simulink model "momentumBasedFlying"  (Simulink 10.2)
settings: Solver=FixedStepAuto  StartTime=0.0  StopTime=Config.simulationTime  FixedStep=Config.tStep  RelTol=1e-3
InitFcn:
  | cd(fileparts(which(bdroot)));
  | initMomentumBasedFlying;
StopFcn:
  | cd(fileparts(which(bdroot)));
  | stopMomentumBasedFlying;
undefined symbols (not defined in the file or in its folder): aerodynamics_config, biasVectorConstraint_feet, Config, confVisualizer, ConstraintMatrix_feet, DiscIntNeverNeededParam, jets_config
libraries: WBToolboxLibrary x85
(part 3 of 4)

== system momentumBasedFlying/iRonCub/Forward Dynamics/old_simulator_subsystem/Compute generalized external wrench and jet thrust/Compute generalized jet wrench ==
  <J_jets> : Inport
  <matrixOfJetAxes> : Inport  Port=2
  jets_input : Inport  Port=3
  Discrete-Time Integrator : DiscreteIntegrator  InitialCondition=Config.initialConditions.jets_thrust  SampleTime=-1  ICPrevOutput=DiscIntNeverNeededParam  ICPrevScaledInput=DiscIntNeverNeededParam
  Discrete-Time Integrator1 : DiscreteIntegrator  SampleTime=-1  ICPrevOutput=DiscIntNeverNeededParam  ICPrevScaledInput=DiscIntNeverNeededParam
  J^T*f : Product  Multiplication=Matrix(*)
  Jet Dynamics : MATLAB Function  TreatAsAtomicUnit=on
  Transpose : Math  Operator=transpose  SignedPower=on  SaturateOnIntegerOverflow=on
  "compute_jet_wrenches " : MATLAB Function  TreatAsAtomicUnit=on
  generalized_jet_wrench : Outport  VectorParamsAs1DForOutWhenUnconnected=off
  jet_intensities : Outport  Port=2  VectorParamsAs1DForOutWhenUnconnected=off
  wires:
  "compute_jet_wrenches "/1(wrenches_vector) -> J^T*f/2  "jet_wrenches_vectors"
  <matrixOfJetAxes>/1 -> "compute_jet_wrenches "/1(matrix_of_jet_axis)
  Transpose/1 -> J^T*f/1  "J_jets_transpose"
  <J_jets>/1 -> Transpose/1
  jets_input/1 -> Jet Dynamics/1(u)
  Discrete-Time Integrator/1 -> jet_intensities/1, "compute_jet_wrenches "/2(jet_intensities), Jet Dynamics/2(jetIntensities)  "jet_intensities"
  J^T*f/1 -> generalized_jet_wrench/1  "generalized_jet_wrench"
  Jet Dynamics/2(jetAccelerationOut) -> Discrete-Time Integrator1/1
  Discrete-Time Integrator1/1 -> Jet Dynamics/3(jetDerivatives)  "jets_velocities"
  Jet Dynamics/1(jetDerivativesOut) -> Discrete-Time Integrator/1

== system momentumBasedFlying/iRonCub/Forward Dynamics/old_simulator_subsystem/Dynamics and Kinematics/Dynamic Quantities ==
  w_H_b : Inport
  w_baseTwist : Inport  Port=2
  jointPos : Inport  Port=3
  jointVel : Inport  Port=4
  GetBiasForces : WBToolboxLibrary/Model/Dynamics/GetBiasForces
      settings: SourceProductName=WholeBodyToolbox
  MassMatrix : WBToolboxLibrary/Model/Dynamics/MassMatrix
      settings: SourceProductName=WholeBodyToolbox
  M : Outport  VectorParamsAs1DForOutWhenUnconnected=off
  "h " : Outport  Port=2  VectorParamsAs1DForOutWhenUnconnected=off
  wires:
  w_H_b/1 -> GetBiasForces/1, MassMatrix/1  "w_H_b"
  w_baseTwist/1 -> GetBiasForces/3
  jointVel/1 -> GetBiasForces/4
  MassMatrix/1 -> M/1
  GetBiasForces/1 -> "h "/1
  jointPos/1 -> GetBiasForces/2, MassMatrix/2

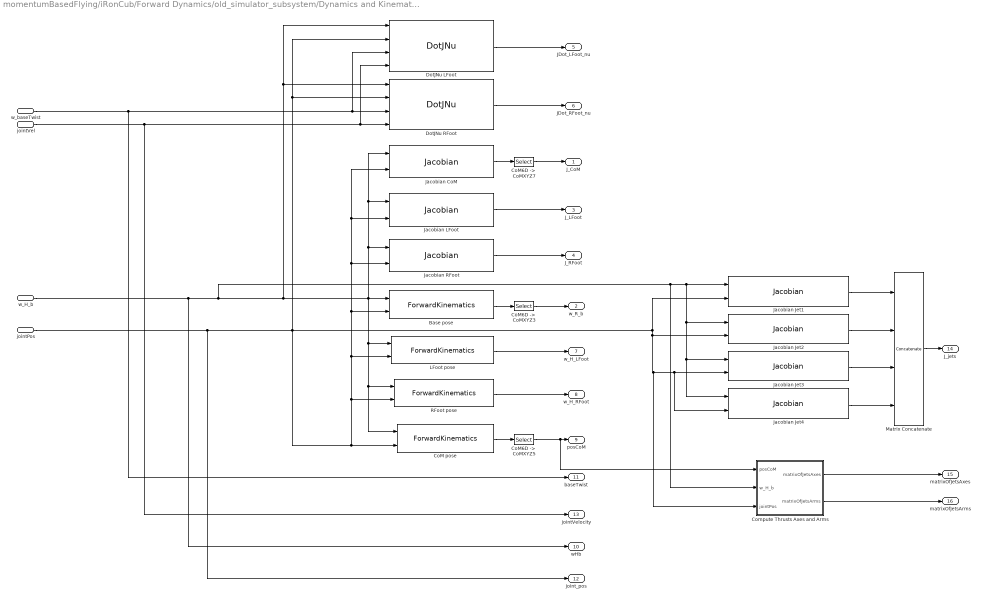
== system momentumBasedFlying/iRonCub/Forward Dynamics/old_simulator_subsystem/Dynamics and Kinematics/Kinematic Quantities ==
  w_H_b : Inport
  w_baseTwist : Inport  Port=2
  jointPos : Inport  Port=3
  jointVel : Inport  Port=4
  Base pose : WBToolboxLibrary/Model/Kinematics/ForwardKinematics  frameName=Frames.BASE_LINK
      settings: SourceProductName=WholeBodyToolbox
  CoM pose : WBToolboxLibrary/Model/Kinematics/ForwardKinematics  frameName=Frames.COM_FRAME
      settings: SourceProductName=WholeBodyToolbox
  "CoM6D ->  CoMXYZ3" : Selector  NumberOfDimensions=2  InputPortWidth=7  IndexOptions=Index vector (dialog),Index vector (dialog)  Indices=[1 2 3],[1 2 3]  OutputSizes=1,1
  "CoM6D ->  CoMXYZ5" : Selector  NumberOfDimensions=2  InputPortWidth=7  IndexOptions=Index vector (dialog),Index vector (dialog)  Indices=[1 2 3],[4]  OutputSizes=1,1
  "CoM6D ->  CoMXYZ7" : Selector  NumberOfDimensions=2  InputPortWidth=7  IndexOptions=Index vector (dialog),Index vector (dialog)  Indices=[1 2 3],[1:6+Config.N_DOF]  OutputSizes=1,1
  Compute Thrusts Axes and Arms : Subsystem
  DotJNu LFoot : WBToolboxLibrary/Model/Jacobians/DotJNu  frameName=Frames.LFOOT_FRAME
      settings: SourceProductName=WholeBodyToolbox
  DotJNu RFoot : WBToolboxLibrary/Model/Jacobians/DotJNu  frameName=Frames.RFOOT_FRAME
      settings: SourceProductName=WholeBodyToolbox
  Jacobian CoM : WBToolboxLibrary/Model/Jacobians/Jacobian  frameName=Frames.COM_FRAME
      settings: SourceProductName=WholeBodyToolbox
  Jacobian Jet1 : WBToolboxLibrary/Model/Jacobians/Jacobian  frameName=Frames.JET1_FRAME
      settings: SourceProductName=WholeBodyToolbox
  Jacobian Jet2 : WBToolboxLibrary/Model/Jacobians/Jacobian  frameName=Frames.JET2_FRAME
      settings: SourceProductName=WholeBodyToolbox
  Jacobian Jet3 : WBToolboxLibrary/Model/Jacobians/Jacobian  frameName=Frames.JET3_FRAME
      settings: SourceProductName=WholeBodyToolbox
  Jacobian Jet4 : WBToolboxLibrary/Model/Jacobians/Jacobian  frameName=Frames.JET4_FRAME
      settings: SourceProductName=WholeBodyToolbox
  Jacobian LFoot : WBToolboxLibrary/Model/Jacobians/Jacobian  frameName=Frames.LFOOT_FRAME
      settings: SourceProductName=WholeBodyToolbox
  Jacobian RFoot : WBToolboxLibrary/Model/Jacobians/Jacobian  frameName=Frames.RFOOT_FRAME
      settings: SourceProductName=WholeBodyToolbox
  LFoot pose : WBToolboxLibrary/Model/Kinematics/ForwardKinematics  frameName=Frames.LFOOT_FRAME
      settings: SourceProductName=WholeBodyToolbox
  Matrix Concatenate : Concatenate  NumInputs=4  Mode=Multidimensional array
  RFoot pose : WBToolboxLibrary/Model/Kinematics/ForwardKinematics  frameName=Frames.RFOOT_FRAME
      settings: SourceProductName=WholeBodyToolbox
  J_CoM : Outport  VectorParamsAs1DForOutWhenUnconnected=off
  w_R_b : Outport  Port=2  VectorParamsAs1DForOutWhenUnconnected=off
  J_LFoot : Outport  Port=3  VectorParamsAs1DForOutWhenUnconnected=off
  J_RFoot : Outport  Port=4  VectorParamsAs1DForOutWhenUnconnected=off
  JDot_LFoot_nu : Outport  Port=5  VectorParamsAs1DForOutWhenUnconnected=off
  JDot_RFoot_nu : Outport  Port=6  VectorParamsAs1DForOutWhenUnconnected=off
  w_H_LFoot : Outport  Port=7  VectorParamsAs1DForOutWhenUnconnected=off
  w_H_RFoot : Outport  Port=8  VectorParamsAs1DForOutWhenUnconnected=off
  posCoM : Outport  Port=9  VectorParamsAs1DForOutWhenUnconnected=off
  wHb : Outport  Port=10
  baseTwist : Outport  Port=11
  joint_pos : Outport  Port=12
  jointVelocity : Outport  Port=13
  J_jets : Outport  Port=14  VectorParamsAs1DForOutWhenUnconnected=off
  matrixOfJetsAxes : Outport  Port=15  VectorParamsAs1DForOutWhenUnconnected=off
  matrixOfJetsArms : Outport  Port=16  VectorParamsAs1DForOutWhenUnconnected=off
  wires:
  CoM pose/1 -> "CoM6D ->  CoMXYZ5"/1
  "CoM6D ->  CoMXYZ3"/1 -> w_R_b/1
  Jacobian CoM/1 -> "CoM6D ->  CoMXYZ7"/1
  Jacobian RFoot/1 -> J_RFoot/1
  Jacobian LFoot/1 -> J_LFoot/1
  DotJNu RFoot/1 -> JDot_RFoot_nu/1
  DotJNu LFoot/1 -> JDot_LFoot_nu/1
  jointVel/1 -> jointVelocity/1, DotJNu RFoot/4, DotJNu LFoot/4
  w_baseTwist/1 -> baseTwist/1, DotJNu LFoot/3, DotJNu RFoot/3
  RFoot pose/1 -> w_H_RFoot/1
  LFoot pose/1 -> w_H_LFoot/1
  Base pose/1 -> "CoM6D ->  CoMXYZ3"/1
  "CoM6D ->  CoMXYZ7"/1 -> J_CoM/1
  Compute Thrusts Axes and Arms/1(matrixOfJetsAxes) -> matrixOfJetsAxes/1
  Compute Thrusts Axes and Arms/2(matrixOfJetsArms) -> matrixOfJetsArms/1
  w_H_b/1 -> Compute Thrusts Axes and Arms/2(w_H_b), Jacobian Jet4/1, Jacobian Jet3/1, Jacobian Jet2/1, Jacobian Jet1/1, DotJNu LFoot/1, DotJNu RFoot/1, Jacobian LFoot/1, Jacobian CoM/1, Jacobian RFoot/1, CoM pose/1, RFoot pose/1, LFoot pose/1, Base pose/1, wHb/1
  Matrix Concatenate/1 -> J_jets/1
  Jacobian Jet3/1 -> Matrix Concatenate/3
  jointPos/1 -> Jacobian Jet4/2, Jacobian Jet3/2, Compute Thrusts Axes and Arms/3(jointPos), Jacobian Jet2/2, Jacobian Jet1/2, LFoot pose/2, Jacobian RFoot/2, Jacobian LFoot/2, Jacobian CoM/2, Base pose/2, RFoot pose/2, CoM pose/2, DotJNu RFoot/2, DotJNu LFoot/2, joint_pos/1
  Jacobian Jet4/1 -> Matrix Concatenate/4
  Jacobian Jet1/1 -> Matrix Concatenate/1
  Jacobian Jet2/1 -> Matrix Concatenate/2
  "CoM6D ->  CoMXYZ5"/1 -> Compute Thrusts Axes and Arms/1(posCoM), posCoM/1

== system momentumBasedFlying/FLYING CONTROLLER (CORE) V2.5/Dynamics and Kinematics/Dynamic Quantities/Momentum and CentroidalMomentum Matrix/CentroidalMomentum Matrix iCub 23/25 DoFs/CMM_base ==
  w_H_b : Inport
  jointPos : Inport  Port=2
  CentroidalMomentum{21..25,31} (6 alike) : WBToolboxLibrary/Model/Dynamics/CentroidalMomentum
      settings: SourceProductName=WholeBodyToolbox
  Constant : Constant  Value=[1,0,0,0,0,0]
  Constant1 : Constant  Value=[0,1,0,0,0,0]
  Constant2 : Constant  Value=zeros(Config.N_DOF,1)
  Constant3 : Constant  Value=[0,0,0,1,0,0]
  Constant37 : Constant  Value=[0,0,1,0,0,0]
  Constant4 : Constant  Value=[0,0,0,0,1,0]
  Constant6 : Constant  Value=[0,0,0,0,0,1]
  Matrix Concatenate : Concatenate  NumInputs=6  Mode=Multidimensional array  ConcatenateDimension=2
  CMM_base : Outport  VectorParamsAs1DForOutWhenUnconnected=off
  wires:
  w_H_b/1 -> CentroidalMomentum31/1, CentroidalMomentum25/1, CentroidalMomentum24/1, CentroidalMomentum23/1, CentroidalMomentum22/1, CentroidalMomentum21/1
  jointPos/1 -> CentroidalMomentum31/2, CentroidalMomentum25/2, CentroidalMomentum24/2, CentroidalMomentum23/2, CentroidalMomentum22/2, CentroidalMomentum21/2
  CentroidalMomentum25/1 -> Matrix Concatenate/5
  Matrix Concatenate/1 -> CMM_base/1
  CentroidalMomentum23/1 -> Matrix Concatenate/3
  CentroidalMomentum24/1 -> Matrix Concatenate/4
  CentroidalMomentum31/1 -> Matrix Concatenate/6
  Constant6/1 -> CentroidalMomentum31/3
  Constant/1 -> CentroidalMomentum21/3
  Constant1/1 -> CentroidalMomentum22/3
  Constant37/1 -> CentroidalMomentum23/3
  Constant2/1 -> CentroidalMomentum21/4, CentroidalMomentum31/4, CentroidalMomentum25/4, CentroidalMomentum24/4, CentroidalMomentum23/4, CentroidalMomentum22/4
  Constant4/1 -> CentroidalMomentum25/3
  Constant3/1 -> CentroidalMomentum24/3
  CentroidalMomentum22/1 -> Matrix Concatenate/2
  CentroidalMomentum21/1 -> Matrix Concatenate/1

== system momentumBasedFlying/FLYING CONTROLLER (CORE) V2.5/Dynamics and Kinematics/Dynamic Quantities/Momentum and CentroidalMomentum Matrix/CentroidalMomentum Matrix iCub 23/25 DoFs/CMM_joints ==
  w_H_b : Inport
  jointPos : Inport  Port=2
  SelMatrix : Inport  Port=3
  CMM Joints Group 1 : Subsystem
  CMM Joints Group 2 : Subsystem
  CMM Joints Group 3 : Subsystem
  CMM Joints Group 4 : Subsystem
  CMM Joints Group 5 : Subsystem
  Matrix Concatenate6 : Concatenate  NumInputs=4  Mode=Multidimensional array  ConcatenateDimension=2
  CMM_joints_from_1_to_20 : Outport  VectorParamsAs1DForOutWhenUnconnected=off
  CMM_group5_25DoFs : Outport  Port=2  VectorParamsAs1DForOutWhenUnconnected=off
  CMM_group5_23DoFs : Outport  Port=3  VectorParamsAs1DForOutWhenUnconnected=off
  wires:
  Matrix Concatenate6/1 -> CMM_joints_from_1_to_20/1
  w_H_b/1 -> CMM Joints Group 1/1(w_H_b), CMM Joints Group 2/1(w_H_b), CMM Joints Group 3/1(w_H_b), CMM Joints Group 4/1(w_H_b), CMM Joints Group 5/1(w_H_b)
  jointPos/1 -> CMM Joints Group 2/2(jointPos), CMM Joints Group 1/2(jointPos), CMM Joints Group 3/2(jointPos), CMM Joints Group 4/2(jointPos), CMM Joints Group 5/2(jointPos)
  SelMatrix/1 -> CMM Joints Group 3/3(SelMatrix), CMM Joints Group 2/3(SelMatrix), CMM Joints Group 1/3(SelMatrix), CMM Joints Group 4/3(SelMatrix), CMM Joints Group 5/3(SelMatrix)
  CMM Joints Group 1/1(CMM_group1) -> Matrix Concatenate6/1
  CMM Joints Group 2/1(CMM_group2) -> Matrix Concatenate6/2
  CMM Joints Group 3/1(CMM_group3) -> Matrix Concatenate6/3
  CMM Joints Group 4/1(CMM_group4) -> Matrix Concatenate6/4
  CMM Joints Group 5/1(CMM_group5_25DoFs) -> CMM_group5_25DoFs/1
  CMM Joints Group 5/2(CMM_group5_23DoFs) -> CMM_group5_23DoFs/1

== system momentumBasedFlying/FLYING CONTROLLER (CORE) V2.5/Dynamics and Kinematics/Dynamic Quantities/Momentum and CentroidalMomentum Matrix/CentroidalMomentum Matrix iCub 23/25 DoFs/Combine CMM ==
  CMM_base : Inport
  CMM_joints_1_20 : Inport  Port=2
  CMM_group5_25DoFs : Inport  Port=3
  CMM_group5_23DoFs : Inport  Port=4
  Matrix Concatenate1 : Concatenate  Mode=Multidimensional array  ConcatenateDimension=2
  Matrix Concatenate2 : Concatenate  Mode=Multidimensional array  ConcatenateDimension=2
  Matrix Concatenate6 : Concatenate  Mode=Multidimensional array  ConcatenateDimension=2
  CMM_25DoFs : Outport  VectorParamsAs1DForOutWhenUnconnected=off
  CMM_23DoFs : Outport  Port=2  VectorParamsAs1DForOutWhenUnconnected=off
  wires:
  Matrix Concatenate2/1 -> CMM_25DoFs/1
  Matrix Concatenate1/1 -> CMM_23DoFs/1
  CMM_group5_23DoFs/1 -> Matrix Concatenate1/2
  CMM_group5_25DoFs/1 -> Matrix Concatenate2/2
  Matrix Concatenate6/1 -> Matrix Concatenate2/1, Matrix Concatenate1/1
  CMM_base/1 -> Matrix Concatenate6/1
  CMM_joints_1_20/1 -> Matrix Concatenate6/2

== system momentumBasedFlying/FLYING CONTROLLER (CORE) V2.5/Flying Controller v2.5/Momentum Control for Flying/QP Solver and Integrate Contact Forces Derivative/Integrate the Contact Forces Derivative/deadZone ==
  u : Inport
  Constant : Constant  Value=Config.sat.deadZoneThreshold
  Deadzone Function : MATLAB Function  TreatAsAtomicUnit=on
  u_cut : Outport  VectorParamsAs1DForOutWhenUnconnected=off
  wires:
  Deadzone Function/1(y) -> u_cut/1
  u/1 -> Deadzone Function/1(u)
  Constant/1 -> Deadzone Function/2(thr)

== system momentumBasedFlying/FLYING CONTROLLER (CORE) V2.5/Flying State Machine/Compute Gains And References/Smooth CoM and Base References/Smooth Reference Orientations/Rotational PID Controller ==
  w_R_b_des : Inport
  gainSmoothingBaseRot : Inport  Port=2
  Compute Rotation Matrix Derivative : MATLAB Function  TreatAsAtomicUnit=on
  Discrete-Time Integrator2 : DiscreteIntegrator  InitialConditionSource=external  InitialCondition=zeros(3,1)  SampleTime=Config.tStep  ICPrevOutput=DiscIntNeverNeededParam  ICPrevScaledInput=DiscIntNeverNeededParam
  "holder " : WBToolboxLibrary/Utilities/holder 
      settings: SourceProductName=WholeBodyToolbox
  w_R_b_des_smooth : Outport  VectorParamsAs1DForOutWhenUnconnected=off
  body_omega_b_des_smooth : Outport  Port=2  VectorParamsAs1DForOutWhenUnconnected=off
  wires:
  "holder "/1 -> Discrete-Time Integrator2/2
  Compute Rotation Matrix Derivative/2(RDot) -> Discrete-Time Integrator2/1
  Discrete-Time Integrator2/1 -> w_R_b_des_smooth/1, Compute Rotation Matrix Derivative/3(w_R_b)
  w_R_b_des/1 -> "holder "/1, Compute Rotation Matrix Derivative/2(w_R_b_des)
  Compute Rotation Matrix Derivative/1(b_omega_b) -> body_omega_b_des_smooth/1
  gainSmoothingBaseRot/1 -> Compute Rotation Matrix Derivative/1(gainSmoothingBaseRot)

== system momentumBasedFlying/iRonCub/Forward Dynamics/old_simulator_subsystem/Dynamics and Kinematics/Kinematic Quantities/Compute Thrusts Axes and Arms ==
  posCoM : Inport
  w_H_b : Inport  Port=2
  jointPos : Inport  Port=3
  Pose Jet 1 : WBToolboxLibrary/Model/Kinematics/ForwardKinematics  frameName=Frames.JET1_FRAME
      settings: SourceProductName=WholeBodyToolbox
  Pose Jet 2 : WBToolboxLibrary/Model/Kinematics/ForwardKinematics  frameName=Frames.JET2_FRAME
      settings: SourceProductName=WholeBodyToolbox
  Pose Jet 3 : WBToolboxLibrary/Model/Kinematics/ForwardKinematics  frameName=Frames.JET3_FRAME
      settings: SourceProductName=WholeBodyToolbox
  Pose Jet 4 : WBToolboxLibrary/Model/Kinematics/ForwardKinematics  frameName=Frames.JET4_FRAME
      settings: SourceProductName=WholeBodyToolbox
  Thrust Axes and Arms : MATLAB Function  TreatAsAtomicUnit=on
  matrixOfJetsAxes : Outport  VectorParamsAs1DForOutWhenUnconnected=off
  matrixOfJetsArms : Outport  Port=2  VectorParamsAs1DForOutWhenUnconnected=off
  wires:
  Pose Jet 2/1 -> Thrust Axes and Arms/2(w_H_J2)
  jointPos/1 -> Pose Jet 1/2, Pose Jet 2/2, Pose Jet 3/2, Pose Jet 4/2
  Pose Jet 1/1 -> Thrust Axes and Arms/1(w_H_J1)
  Pose Jet 3/1 -> Thrust Axes and Arms/3(w_H_J3)
  Pose Jet 4/1 -> Thrust Axes and Arms/4(w_H_J4)
  Thrust Axes and Arms/1(matrixOfJetsAxes) -> matrixOfJetsAxes/1
  Thrust Axes and Arms/2(matrixOfJetsArms) -> matrixOfJetsArms/1
  w_H_b/1 -> Pose Jet 4/1, Pose Jet 3/1, Pose Jet 2/1, Pose Jet 1/1
  posCoM/1 -> Thrust Axes and Arms/5(posCoM)

== system momentumBasedFlying/FLYING CONTROLLER (CORE) V2.5/Dynamics and Kinematics/Dynamic Quantities/Momentum and CentroidalMomentum Matrix/CentroidalMomentum Matrix iCub 23/25 DoFs/CMM_joints/CMM Joints Group 1 ==
  w_H_b : Inport
  jointPos : Inport  Port=2
  SelMatrix : Inport  Port=3
  CentroidalMomentum{1..4,16} (5 alike) : WBToolboxLibrary/Model/Dynamics/CentroidalMomentum
      settings: SourceProductName=WholeBodyToolbox
  Constant : Constant  Value=zeros(6,1)
  Constant1 : Constant
  MATLAB Function : MATLAB Function  TreatAsAtomicUnit=on
  Matrix Concatenate6 : Concatenate  NumInputs=5  Mode=Multidimensional array  ConcatenateDimension=2
  CMM_group1 : Outport  VectorParamsAs1DForOutWhenUnconnected=off
  wires:
  Constant/1 -> CentroidalMomentum4/3, CentroidalMomentum3/3, CentroidalMomentum1/3, CentroidalMomentum16/3, CentroidalMomentum2/3
  CentroidalMomentum2/1 -> Matrix Concatenate6/3
  CentroidalMomentum1/1 -> Matrix Concatenate6/2
  CentroidalMomentum3/1 -> Matrix Concatenate6/4
  CentroidalMomentum16/1 -> Matrix Concatenate6/1
  w_H_b/1 -> CentroidalMomentum1/1, CentroidalMomentum2/1, CentroidalMomentum3/1, CentroidalMomentum4/1, CentroidalMomentum16/1
  CentroidalMomentum4/1 -> Matrix Concatenate6/5
  Matrix Concatenate6/1 -> CMM_group1/1
  MATLAB Function/1(v1) -> CentroidalMomentum16/4
  MATLAB Function/2(v2) -> CentroidalMomentum1/4
  MATLAB Function/3(v3) -> CentroidalMomentum2/4
  MATLAB Function/4(v4) -> CentroidalMomentum3/4
  MATLAB Function/5(v5) -> CentroidalMomentum4/4
  SelMatrix/1 -> MATLAB Function/1(SelMatrix)
  Constant1/1 -> MATLAB Function/2(groupNumber)
  jointPos/1 -> MATLAB Function/3(jointPos), CentroidalMomentum4/2, CentroidalMomentum3/2, CentroidalMomentum2/2, CentroidalMomentum16/2, CentroidalMomentum1/2

== system momentumBasedFlying/FLYING CONTROLLER (CORE) V2.5/Dynamics and Kinematics/Dynamic Quantities/Momentum and CentroidalMomentum Matrix/CentroidalMomentum Matrix iCub 23/25 DoFs/CMM_joints/CMM Joints Group 2 ==
  w_H_b : Inport
  jointPos : Inport  Port=2
  SelMatrix : Inport  Port=3
  CentroidalMomentum{1..4,16} (5 alike) : WBToolboxLibrary/Model/Dynamics/CentroidalMomentum
      settings: SourceProductName=WholeBodyToolbox
  Constant : Constant  Value=zeros(6,1)
  Constant1 : Constant  Value=2
  MATLAB Function : MATLAB Function  TreatAsAtomicUnit=on
  Matrix Concatenate6 : Concatenate  NumInputs=5  Mode=Multidimensional array  ConcatenateDimension=2
  CMM_group2 : Outport  VectorParamsAs1DForOutWhenUnconnected=off
  wires:
  Constant/1 -> CentroidalMomentum4/3, CentroidalMomentum3/3, CentroidalMomentum1/3, CentroidalMomentum16/3, CentroidalMomentum2/3
  CentroidalMomentum2/1 -> Matrix Concatenate6/3
  CentroidalMomentum1/1 -> Matrix Concatenate6/2
  CentroidalMomentum3/1 -> Matrix Concatenate6/4
  CentroidalMomentum16/1 -> Matrix Concatenate6/1
  w_H_b/1 -> CentroidalMomentum1/1, CentroidalMomentum2/1, CentroidalMomentum3/1, CentroidalMomentum4/1, CentroidalMomentum16/1
  CentroidalMomentum4/1 -> Matrix Concatenate6/5
  Matrix Concatenate6/1 -> CMM_group2/1
  MATLAB Function/1(v1) -> CentroidalMomentum16/4
  MATLAB Function/2(v2) -> CentroidalMomentum1/4
  MATLAB Function/3(v3) -> CentroidalMomentum2/4
  MATLAB Function/4(v4) -> CentroidalMomentum3/4
  MATLAB Function/5(v5) -> CentroidalMomentum4/4
  SelMatrix/1 -> MATLAB Function/1(SelMatrix)
  Constant1/1 -> MATLAB Function/2(groupNumber)
  jointPos/1 -> MATLAB Function/3(jointPos), CentroidalMomentum4/2, CentroidalMomentum3/2, CentroidalMomentum2/2, CentroidalMomentum16/2, CentroidalMomentum1/2

== system momentumBasedFlying/FLYING CONTROLLER (CORE) V2.5/Dynamics and Kinematics/Dynamic Quantities/Momentum and CentroidalMomentum Matrix/CentroidalMomentum Matrix iCub 23/25 DoFs/CMM_joints/CMM Joints Group 3 ==
  w_H_b : Inport
  jointPos : Inport  Port=2
  SelMatrix : Inport  Port=3
  CentroidalMomentum{1..4,16} (5 alike) : WBToolboxLibrary/Model/Dynamics/CentroidalMomentum
      settings: SourceProductName=WholeBodyToolbox
  Constant : Constant  Value=zeros(6,1)
  Constant1 : Constant  Value=3
  MATLAB Function : MATLAB Function  TreatAsAtomicUnit=on
  Matrix Concatenate6 : Concatenate  NumInputs=5  Mode=Multidimensional array  ConcatenateDimension=2
  CMM_group3 : Outport  VectorParamsAs1DForOutWhenUnconnected=off
  wires:
  Constant/1 -> CentroidalMomentum4/3, CentroidalMomentum3/3, CentroidalMomentum1/3, CentroidalMomentum16/3, CentroidalMomentum2/3
  CentroidalMomentum2/1 -> Matrix Concatenate6/3
  CentroidalMomentum1/1 -> Matrix Concatenate6/2
  CentroidalMomentum3/1 -> Matrix Concatenate6/4
  CentroidalMomentum16/1 -> Matrix Concatenate6/1
  w_H_b/1 -> CentroidalMomentum1/1, CentroidalMomentum2/1, CentroidalMomentum3/1, CentroidalMomentum4/1, CentroidalMomentum16/1
  CentroidalMomentum4/1 -> Matrix Concatenate6/5
  Matrix Concatenate6/1 -> CMM_group3/1
  MATLAB Function/1(v1) -> CentroidalMomentum16/4
  MATLAB Function/2(v2) -> CentroidalMomentum1/4
  MATLAB Function/3(v3) -> CentroidalMomentum2/4
  MATLAB Function/4(v4) -> CentroidalMomentum3/4
  MATLAB Function/5(v5) -> CentroidalMomentum4/4
  SelMatrix/1 -> MATLAB Function/1(SelMatrix)
  Constant1/1 -> MATLAB Function/2(groupNumber)
  jointPos/1 -> MATLAB Function/3(jointPos), CentroidalMomentum4/2, CentroidalMomentum3/2, CentroidalMomentum2/2, CentroidalMomentum16/2, CentroidalMomentum1/2

== system momentumBasedFlying/FLYING CONTROLLER (CORE) V2.5/Dynamics and Kinematics/Dynamic Quantities/Momentum and CentroidalMomentum Matrix/CentroidalMomentum Matrix iCub 23/25 DoFs/CMM_joints/CMM Joints Group 4 ==
  w_H_b : Inport
  jointPos : Inport  Port=2
  SelMatrix : Inport  Port=3
  CentroidalMomentum{1..4,16} (5 alike) : WBToolboxLibrary/Model/Dynamics/CentroidalMomentum
      settings: SourceProductName=WholeBodyToolbox
  Constant : Constant  Value=zeros(6,1)
  Constant1 : Constant  Value=4
  MATLAB Function : MATLAB Function  TreatAsAtomicUnit=on
  Matrix Concatenate6 : Concatenate  NumInputs=5  Mode=Multidimensional array  ConcatenateDimension=2
  CMM_group4 : Outport  VectorParamsAs1DForOutWhenUnconnected=off
  wires:
  Constant/1 -> CentroidalMomentum4/3, CentroidalMomentum3/3, CentroidalMomentum1/3, CentroidalMomentum16/3, CentroidalMomentum2/3
  CentroidalMomentum2/1 -> Matrix Concatenate6/3
  CentroidalMomentum1/1 -> Matrix Concatenate6/2
  CentroidalMomentum3/1 -> Matrix Concatenate6/4
  CentroidalMomentum16/1 -> Matrix Concatenate6/1
  w_H_b/1 -> CentroidalMomentum1/1, CentroidalMomentum2/1, CentroidalMomentum3/1, CentroidalMomentum4/1, CentroidalMomentum16/1
  CentroidalMomentum4/1 -> Matrix Concatenate6/5
  Matrix Concatenate6/1 -> CMM_group4/1
  MATLAB Function/1(v1) -> CentroidalMomentum16/4
  MATLAB Function/2(v2) -> CentroidalMomentum1/4
  MATLAB Function/3(v3) -> CentroidalMomentum2/4
  MATLAB Function/4(v4) -> CentroidalMomentum3/4
  MATLAB Function/5(v5) -> CentroidalMomentum4/4
  SelMatrix/1 -> MATLAB Function/1(SelMatrix)
  Constant1/1 -> MATLAB Function/2(groupNumber)
  jointPos/1 -> MATLAB Function/3(jointPos), CentroidalMomentum4/2, CentroidalMomentum3/2, CentroidalMomentum2/2, CentroidalMomentum16/2, CentroidalMomentum1/2

== system momentumBasedFlying/FLYING CONTROLLER (CORE) V2.5/Dynamics and Kinematics/Dynamic Quantities/Momentum and CentroidalMomentum Matrix/CentroidalMomentum Matrix iCub 23/25 DoFs/CMM_joints/CMM Joints Group 5 ==
  w_H_b : Inport
  jointPos : Inport  Port=2
  SelMatrix : Inport  Port=3
  CentroidalMomentum{1..4,16} (5 alike) : WBToolboxLibrary/Model/Dynamics/CentroidalMomentum
      settings: SourceProductName=WholeBodyToolbox
  Constant : Constant  Value=zeros(6,1)
  Constant1 : Constant  Value=5
  MATLAB Function : MATLAB Function  TreatAsAtomicUnit=on
  Matrix Concatenate1 : Concatenate  Mode=Multidimensional array  ConcatenateDimension=2
  Matrix Concatenate2 : Concatenate  Mode=Multidimensional array  ConcatenateDimension=2
  Matrix Concatenate6 : Concatenate  NumInputs=3  Mode=Multidimensional array  ConcatenateDimension=2
  CMM_group5_25DoFs : Outport  VectorParamsAs1DForOutWhenUnconnected=off
  CMM_group5_23DoFs : Outport  Port=2  VectorParamsAs1DForOutWhenUnconnected=off
  wires:
  Constant/1 -> CentroidalMomentum4/3, CentroidalMomentum3/3, CentroidalMomentum1/3, CentroidalMomentum16/3, CentroidalMomentum2/3
  CentroidalMomentum2/1 -> Matrix Concatenate6/3
  CentroidalMomentum1/1 -> Matrix Concatenate6/2
  jointPos/1 -> CentroidalMomentum4/2, MATLAB Function/3(jointPos), CentroidalMomentum3/2, CentroidalMomentum2/2, CentroidalMomentum16/2, CentroidalMomentum1/2
  CentroidalMomentum16/1 -> Matrix Concatenate6/1
  w_H_b/1 -> CentroidalMomentum1/1, CentroidalMomentum2/1, CentroidalMomentum3/1, CentroidalMomentum4/1, CentroidalMomentum16/1
  MATLAB Function/1(v1) -> CentroidalMomentum16/4
  MATLAB Function/2(v2) -> CentroidalMomentum1/4
  MATLAB Function/3(v3) -> CentroidalMomentum2/4
  MATLAB Function/4(v4) -> CentroidalMomentum3/4
  MATLAB Function/5(v5) -> CentroidalMomentum4/4
  SelMatrix/1 -> MATLAB Function/1(SelMatrix)
  Constant1/1 -> MATLAB Function/2(groupNumber)
  Matrix Concatenate6/1 -> CMM_group5_23DoFs/1, Matrix Concatenate2/1
  CentroidalMomentum4/1 -> Matrix Concatenate1/2
  CentroidalMomentum3/1 -> Matrix Concatenate1/1
  Matrix Concatenate1/1 -> Matrix Concatenate2/2
  Matrix Concatenate2/1 -> CMM_group5_25DoFs/1

== matlab function Visualizer/Task and Base Frame Kinematics/MATLAB Function1 ==
  data: RPY_Corr output double; rollPitchYaw input double
function RPY_Corr = correctYawAngleFCN(rollPitchYaw)

    RPY_Corr = correctYawAngle(rollPitchYaw);

end

== matlab function iRonCub/Forward Dynamics/old_simulator_subsystem/MATLAB Function1 ==
  data: base_linear_velocity output double; mass_matrix input double; bias_forces input double; joints_torque input double; generalized_ext_wrench input double; base_velocity input double; joints_velocity input double; JLeft_frameJac input double; JRight_frameJac input double; JDot_nu_LFOOT input double; JDot_nu_RFOOT input double; H_LFOOT input double; H_RFOOT input double; Config parameter double; omega_b output double; joints_velocity output double; dot_v_b output double; dot_omega_b output double; joint_acceleration output double; contact_detected output double; wrench_left_foot output double; wrench_right_foot output double
function [base_linear_velocity, omega_b, joints_velocity, dot_v_b, dot_omega_b, joint_acceleration, ...
    contact_detected, wrench_left_foot, wrench_right_foot] = ...
    forward_and_contact_dynamics(mass_matrix, bias_forces, joints_torque, generalized_ext_wrench, ...
    base_velocity, joints_velocity, JLeft_frameJac, JRight_frameJac, JDot_nu_LFOOT, JDot_nu_RFOOT, H_LFOOT, H_RFOOT, Config)

[base_linear_velocity, omega_b, joints_velocity, dot_v_b, dot_omega_b, joint_acceleration, ...
    contact_detected, wrench_left_foot, wrench_right_foot] = ...
    forward_and_contact_dynamics(mass_matrix, bias_forces, joints_torque, generalized_ext_wrench, ...
    base_velocity, joints_velocity, JLeft_frameJac, JRight_frameJac, JDot_nu_LFOOT, JDot_nu_RFOOT, H_LFOOT, H_RFOOT, Config);
end

== matlab function Visualizer/Task and Base Frame Kinematics/MATLAB Function3 ==
  data: RPY_Corr output double; rollPitchYaw input double
function RPY_Corr = correctYawAngleFCN(rollPitchYaw)

    RPY_Corr = correctYawAngle(rollPitchYaw);

end

== matlab function Visualizer/Task and Base Frame Kinematics/Get RPY from rotation matrix  ==
  data: w_R_b input double; rollPitchYaw output double
function rollPitchYaw = rollPitchYawFromRotationFCN(w_R_b)

rollPitchYaw = wbc.rollPitchYawFromRotation(w_R_b);

end

== matlab function FLYING CONTROLLER (CORE) V2.5/Dynamics and Kinematics/Dynamic Quantities/Compute Centroidal Inertia/Compute Centroidal Inertia ==
  data: M input double; w_I_c output double; posCoM input double; posBase input double
function w_I_c = getCentrInertiaFCN(M, posCoM, posBase)

    w_I_c = getCentrInertia(M, posCoM, posBase);
end

== matlab function Visualizer/Task and Base Frame Kinematics/Get RPY from rotation matrix ==
  data: w_R_b input double; rollPitchYaw output double
function rollPitchYaw = rollPitchYawFromRotationFCN(w_R_b)

rollPitchYaw = wbc.rollPitchYawFromRotation(w_R_b);

end

== matlab function Visualizer/Task and Base Frame Kinematics/Get RPY error norm ==
  data: rot_err input double; rotErr_norm output double
function rotErr_norm = normFCN(rot_err)

rotErr_norm = norm(rot_err);

end

== matlab function FLYING CONTROLLER (CORE) V2.5/Dynamics and Kinematics/Dynamic Quantities/Momentum and CentroidalMomentum Matrix/CentroidalMomentum Matrix iCub 23//25 DoFs/Select CMM 23 or 25 ==
  data: CMM_25 input double; N_DOF input double; CMM output double; CMM_23 input double
function CMM = selectCMM_23_25_FCN(CMM_25, N_DOF, CMM_23)

    CMM = CMM_25;
    
    if N_DOF < 25
        
        % dynamic sizing of CMM not allowed
        CMM = [CMM_23, zeros(size(CMM,1),2)];
    end
end

== matlab function FLYING CONTROLLER (CORE) V2.5/Flying State Machine/Take Off//Landing State Detector/MATLAB Function ==
  data: wrench_l input double; feetContactIsActive output double; wrench_r input double; Config parameter double; robotIsLanded output double; oneFootIsInContact output double
function [feetContactIsActive, robotIsLanded, oneFootIsInContact] = feetContactActivationFCN(wrench_l, wrench_r, Config)

    [feetContactIsActive, robotIsLanded, oneFootIsInContact] = feetContactActivation(wrench_l, wrench_r, Config);
end

== matlab function Visualizer/Task and Base Frame Kinematics/MATLAB Function2 ==
  data: RPY_Corr output double; rollPitchYaw input double
function RPY_Corr = correctYawAngleFCN(rollPitchYaw)

    RPY_Corr = correctYawAngle(rollPitchYaw);

end

== matlab function FLYING CONTROLLER (CORE) V2.5/Flying Controller v2.5/Joint Torque Control for Flying/Torque Derivative Saturation/Saturate Torque Derivative ==
  data: u input double; uSat output double; u_0 input double; tStep input double; uDotMax input double
function uSat = saturateInputDerivativeFCN(u, u_0, tStep, uDotMax)

    uSat = wbc.saturateInputDerivative(u, u_0, tStep, uDotMax);
end

== matlab function JoyStick Commands/Replace Joystick with Native GUI ==
  data: gui_input input double; joyButtons output double; joyAxes output double
function [joyButtons,joyAxes] = fromGuiToJoystickFCN(gui_input)

    [joyButtons,joyAxes] = fromGuiToJoystick(gui_input);
end

== matlab function FLYING CONTROLLER (CORE) V2.5/Get System State/Change Contact Forces Representation/Change Contact Forces Representation ==
  data: contactForces_WBD input double; mixed_f_l_sole output double; w_R_l_sole input double; w_R_r_sole input double; mixed_f_r_sole output double
function [mixed_f_l_sole, mixed_f_r_sole] = fromBodyFrameToMixed_contactForcesFCN(contactForces_WBD, w_R_l_sole, w_R_r_sole)

    [mixed_f_l_sole, mixed_f_r_sole] = fromBodyFrameToMixed_contactForces(contactForces_WBD, w_R_l_sole, w_R_r_sole);
end

== matlab function FLYING CONTROLLER (CORE) V2.5/Flying State Machine/Compute Gains And References/Compute Gains/Diagonalize ==
  data: k input double; K output double
function K = diagonalMatrixFromVectorFCN(k)

    K = wbc.diagonalMatrixFromVector(k);
end

== matlab function FLYING CONTROLLER (CORE) V2.5/Flying State Machine/Compute Gains And References/Compute Gains/Diagonalize1 ==
  data: k input double; K output double
function K = diagonalMatrixFromVectorFCN(k)

    K = wbc.diagonalMatrixFromVector(k);
end

== matlab function FLYING CONTROLLER (CORE) V2.5/Flying State Machine/Compute Gains And References/Compute Gains/Diagonalize2 ==
  data: k input double; K output double
function K = diagonalMatrixFromVectorFCN(k)

    K = wbc.diagonalMatrixFromVector(k);
end

== matlab function FLYING CONTROLLER (CORE) V2.5/Flying Controller v2.5/Momentum Control for Flying/Momentum Control/Flying Controller Momentum FCN  ==
  data: jointPos input double; w_baseTwist input double; jetsIntensities input double; J_jets input double; J_CoM input double; J_LFoot input double; J_RFoot input double; posCoM input double; w_R_b input double; w_H_LFoot input double; w_H_RFoot input double; matrixOfJetsAxes input double; matrixOfJetsArms input double; w_I_c input double; L input double; M input double; CMM input double; pos_vel_acc_jerk_CoM_des input double; rot_vel_acc_jerk_base_des input double size=[3,6]; jointPos_des input double; KP_momentum input double; KD_momentum input double; KP_postural input double; feetContactIsActive input double; decreaseMaxFootVerticalForce input double; increaseMinFootVerticalForce input double; robotIsLanded input double; HessianMatrixQP output double; gVectorQP output double; lowerBoundQP output double; upperBoundQP output double; L_des output double size=[6,1]; LDot_estimated output double size=[6,1]; verifyAngMomAndInertia output double; contactForces_hat input double; Config parameter double
function [HessianMatrixQP, gVectorQP, lowerBoundQP, upperBoundQP, L_des, LDot_estimated, verifyAngMomAndInertia] = ...
             flyingMomentumControlFCN(jointPos, w_baseTwist, jetsIntensities, J_jets, J_CoM, J_LFoot, J_RFoot, posCoM, w_R_b, w_H_LFoot, ...
                                      w_H_RFoot, matrixOfJetsAxes, matrixOfJetsArms, w_I_c, L, M, CMM, pos_vel_acc_jerk_CoM_des, ....
                                      rot_vel_acc_jerk_base_des, jointPos_des, KP_momentum, KD_momentum, KP_postural, feetContactIsActive, ...
                                      decreaseMaxFootVerticalForce, increaseMinFootVerticalForce, robotIsLanded, contactForces_hat, Config)
                               
    [HessianMatrixQP, gVectorQP, lowerBoundQP, upperBoundQP, L_des, LDot_estimated , verifyAngMomAndInertia] = ...
        flyingMomentumControl(jointPos, w_baseTwist, jetsIntensities, J_jets, J_CoM, J_LFoot, J_RFoot, posCoM, w_R_b, w_H_LFoot, ...
                              w_H_RFoot, matrixOfJetsAxes, matrixOfJetsArms, w_I_c, L, M, CMM, pos_vel_acc_jerk_CoM_des, ....
                              rot_vel_acc_jerk_base_des, jointPos_des, KP_momentum, KD_momentum, KP_postural, feetContactIsActive, ...
                               decreaseMaxFootVerticalForce, increaseMinFootVerticalForce, robotIsLanded, contactForces_hat, Config);
end

== matlab function FLYING CONTROLLER (CORE) V2.5/Flying Controller v2.5/Joint Torque Control for Flying/torqueControlFCN ==
  data: M input double; h input double; J_jets input double; J_LFoot input double; J_RFoot input double; JDot_LFoot_nu input double; JDot_RFoot_nu input double; w_H_LFoot input double; w_H_RFoot input double; matrixOfJetsAxes input double; ConstraintsMatrix_feet input double; biasVectorConstraint_feet input double; jetsIntensities input double; stateVel input double; jointVel_star input double; contactForces_star input double; KI_torqueControl input double; KP_torqueControl input double; feetContactIsActive input double; activateEqConstrTorqueControl input double; robotIsLanded input double; jointPos_err input double; Hessian output double; Config parameter double; gradient output double; ConstraintMatrix_inequality output double; biasVectorConstraint_inequality output double; jointVel_err output double
function [Hessian, gradient, ConstraintMatrix_inequality, biasVectorConstraint_inequality, jointVel_err] =  ... 
             flyingTorqueControlFCN(M, h, J_jets, J_LFoot, J_RFoot, JDot_LFoot_nu, JDot_RFoot_nu, w_H_LFoot, w_H_RFoot, matrixOfJetsAxes, ...
                                    ConstraintsMatrix_feet, biasVectorConstraint_feet, jetsIntensities, stateVel, jointVel_star, contactForces_star, ...
                                    KI_torqueControl, KP_torqueControl, feetContactIsActive, activateEqConstrTorqueControl, robotIsLanded, jointPos_err, Config)
                                      
    [Hessian, gradient, ConstraintMatrix_inequality, biasVectorConstraint_inequality, jointVel_err] =  ... 
        flyingTorqueControl(M, h, J_jets, J_LFoot, J_RFoot, JDot_LFoot_nu, JDot_RFoot_nu, w_H_LFoot, w_H_RFoot, matrixOfJetsAxes, ...
                            ConstraintsMatrix_feet, biasVectorConstraint_feet, jetsIntensities, stateVel, jointVel_star, contactForces_star, ...
                            KI_torqueControl, KP_torqueControl, feetContactIsActive, activateEqConstrTorqueControl, robotIsLanded, jointPos_err, Config);           
end

== matlab function FLYING CONTROLLER (CORE) V2.5/Flying State Machine/Compute Gains And References/Compute Gains/Diagonalize3 ==
  data: k input double; K output double
function K = diagonalMatrixFromVectorFCN(k)

    K = wbc.diagonalMatrixFromVector(k);
end

== matlab function FLYING CONTROLLER (CORE) V2.5/Dynamics and Kinematics/Kinematic Quantities/Compute Thrusts Axes and Arms/Thrust Axes and Arms ==
  data: w_H_J1 input double; matrixOfJetsAxes output double; w_H_J2 input double; w_H_J3 input double; w_H_J4 input double; posCoM input double; matrixOfJetsArms output double; Config parameter double
function [matrixOfJetsAxes, matrixOfJetsArms] = computeJetsAxesAndArmsFCN(w_H_J1, w_H_J2, w_H_J3, w_H_J4, posCoM, Config)

    [matrixOfJetsAxes, matrixOfJetsArms] = computeJetsAxesAndArms(w_H_J1, w_H_J2, w_H_J3, w_H_J4, posCoM, Config);
end

== matlab function FLYING CONTROLLER (CORE) V2.5/Flying State Machine/Compute Gains And References/Compute Gains/Diagonalize4 ==
  data: k input double; K output double
function K = diagonalMatrixFromVectorFCN(k)

    K = wbc.diagonalMatrixFromVector(k);
end

== matlab function FLYING CONTROLLER (CORE) V2.5/Flying Controller v2.5/Momentum Control for Flying/QP Solver and Integrate Contact Forces Derivative/Integrate the Contact Forces Derivative/deadZone/Deadzone Function ==
  data: u input double; y output double; thr input double
function y = deadZoneFCN(u, thr)

    y = wbc.deadZone(u, thr);
end

== matlab function FLYING CONTROLLER (CORE) V2.5/Flying State Machine/Take Off//Landing State Detector/Vertical Forces Control ==
  data: joyButtons input double; decreaseMaxFootVerticalForce output double; increaseMinFootVerticalForce output double; activateEqConstrTorqueControl output double
function [decreaseMaxFootVerticalForce, increaseMinFootVerticalForce, activateEqConstrTorqueControl] = verticalForcesControlFCN(joyButtons)

    [decreaseMaxFootVerticalForce, increaseMinFootVerticalForce, activateEqConstrTorqueControl] = verticalForcesControl(joyButtons);
end

== matlab function FLYING CONTROLLER (CORE) V2.5/Dynamics and Kinematics/Dynamic Quantities/Momentum and CentroidalMomentum Matrix/CentroidalMomentum Matrix iCub 23//25 DoFs/CMM_joints/CMM Joints Group 1/MATLAB Function ==
  data: SelMatrix input double; v1 output double; groupNumber input double; v2 output double; v3 output double; v4 output double; v5 output double; jointPos input double
function [v1,v2,v3,v4,v5] = selectFiveMatrixColumns(SelMatrix,groupNumber,jointPos)
        
    ndof = length(jointPos);
    
    v1   = SelMatrix((groupNumber-1)*5 + 1,1:ndof);
    v2   = SelMatrix((groupNumber-1)*5 + 2,1:ndof);
    v3   = SelMatrix((groupNumber-1)*5 + 3,1:ndof);
    v4   = SelMatrix((groupNumber-1)*5 + 4,1:ndof);
    v5   = SelMatrix((groupNumber-1)*5 + 5,1:ndof);
end

== matlab function FLYING CONTROLLER (CORE) V2.5/Dynamics and Kinematics/Dynamic Quantities/Momentum and CentroidalMomentum Matrix/CentroidalMomentum Matrix iCub 23//25 DoFs/CMM_joints/CMM Joints Group 2/MATLAB Function ==
  data: SelMatrix input double; v1 output double; groupNumber input double; v2 output double; v3 output double; v4 output double; v5 output double; jointPos input double
function [v1,v2,v3,v4,v5] = selectFiveMatrixColumns(SelMatrix,groupNumber,jointPos)
        
    ndof = length(jointPos);
    
    v1   = SelMatrix((groupNumber-1)*5 + 1,1:ndof);
    v2   = SelMatrix((groupNumber-1)*5 + 2,1:ndof);
    v3   = SelMatrix((groupNumber-1)*5 + 3,1:ndof);
    v4   = SelMatrix((groupNumber-1)*5 + 4,1:ndof);
    v5   = SelMatrix((groupNumber-1)*5 + 5,1:ndof);
end

== matlab function FLYING CONTROLLER (CORE) V2.5/Dynamics and Kinematics/Dynamic Quantities/Momentum and CentroidalMomentum Matrix/CentroidalMomentum Matrix iCub 23//25 DoFs/CMM_joints/CMM Joints Group 3/MATLAB Function ==
  data: SelMatrix input double; v1 output double; groupNumber input double; v2 output double; v3 output double; v4 output double; v5 output double; jointPos input double
function [v1,v2,v3,v4,v5] = selectFiveMatrixColumns(SelMatrix,groupNumber,jointPos)
        
    ndof = length(jointPos);
    
    v1   = SelMatrix((groupNumber-1)*5 + 1,1:ndof);
    v2   = SelMatrix((groupNumber-1)*5 + 2,1:ndof);
    v3   = SelMatrix((groupNumber-1)*5 + 3,1:ndof);
    v4   = SelMatrix((groupNumber-1)*5 + 4,1:ndof);
    v5   = SelMatrix((groupNumber-1)*5 + 5,1:ndof);
end

== matlab function FLYING CONTROLLER (CORE) V2.5/Dynamics and Kinematics/Dynamic Quantities/Momentum and CentroidalMomentum Matrix/CentroidalMomentum Matrix iCub 23//25 DoFs/CMM_joints/CMM Joints Group 4/MATLAB Function ==
  data: SelMatrix input double; v1 output double; groupNumber input double; v2 output double; v3 output double; v4 output double; v5 output double; jointPos input double
function [v1,v2,v3,v4,v5] = selectFiveMatrixColumns(SelMatrix,groupNumber,jointPos)
        
    ndof = length(jointPos);
    
    v1   = SelMatrix((groupNumber-1)*5 + 1,1:ndof);
    v2   = SelMatrix((groupNumber-1)*5 + 2,1:ndof);
    v3   = SelMatrix((groupNumber-1)*5 + 3,1:ndof);
    v4   = SelMatrix((groupNumber-1)*5 + 4,1:ndof);
    v5   = SelMatrix((groupNumber-1)*5 + 5,1:ndof);
end

== matlab function FLYING CONTROLLER (CORE) V2.5/Dynamics and Kinematics/Dynamic Quantities/Momentum and CentroidalMomentum Matrix/CentroidalMomentum Matrix iCub 23//25 DoFs/CMM_joints/CMM Joints Group 5/MATLAB Function ==
  data: SelMatrix input double; v1 output double; groupNumber input double; v2 output double; v3 output double; v4 output double; v5 output double; jointPos input double
function [v1,v2,v3,v4,v5] = selectFiveMatrixColumns(SelMatrix,groupNumber,jointPos)
        
    ndof = length(jointPos);
    
    v1   = SelMatrix((groupNumber-1)*5 + 1,1:ndof);
    v2   = SelMatrix((groupNumber-1)*5 + 2,1:ndof);
    v3   = SelMatrix((groupNumber-1)*5 + 3,1:ndof);
    v4   = SelMatrix((groupNumber-1)*5 + 4,1:ndof);
    v5   = SelMatrix((groupNumber-1)*5 + 5,1:ndof);
end

== matlab function FLYING CONTROLLER (CORE) V2.5/Dynamics and Kinematics/Dynamic Quantities/Momentum and CentroidalMomentum Matrix/CentroidalMomentum Matrix iCub 23//25 DoFs/Selector Matrix ==
  data: ROBOT_DOF input double; SelMatrix output double; SelMatrix_0 input double
function SelMatrix = updateSelectorMatrix(ROBOT_DOF, SelMatrix_0)
    SelMatrix = blkdiag(SelMatrix_0, zeros(2));
end

== matlab function FLYING CONTROLLER (CORE) V2.5/Flying Controller v2.5/Momentum Control for Flying/QP Solver and Integrate Contact Forces Derivative/Integrate the Contact Forces Derivative/Select Integrator Initial Condition ==
  data: feetContactIsActive input double; contactForces input double; contactForces_0 output double
function contactForces_0 = selectInitContactForcesFCN(feetContactIsActive, contactForces)

    contactForces_0 = selectInitContactForces(feetContactIsActive, contactForces);
end

== matlab function FLYING CONTROLLER (CORE) V2.5/Flying Controller v2.5/Momentum Control for Flying/extendedKalmanFilter4jets/EKF_jet1/EKF  ==
  data: x input double; input input double; measurement input double; xDot output double; P input double; Config parameter double; Pdot output double
function [xDot, Pdot] = extendedKalmanFilterFNC(x, input, measurement, P, Config)

[xDot, Pdot] = extKalmanFilter(x, input, Config.jetC_P100, P, measurement, Config);

== matlab function FLYING CONTROLLER (CORE) V2.5/Flying Controller v2.5/Momentum Control for Flying/extendedKalmanFilter4jets/EKF_jet1/splitVector ==
  data: x input double; x1 output double; x2 output double
function [x1, x2] = fcn(x)
x1 = x(1);
x2 = x(2);

== matlab function iRonCub/Forward Dynamics/old_simulator_subsystem/Compute generalized external wrench and jet thrust/Compute generalized jet wrench/Jet Dynamics ==
  data: u input double; jetDerivativesOut output double; jetIntensities input double size=[4,1]; jetDerivatives input double size=[4,1]; Config parameter double; jetAccelerationOut output double
function [jetDerivativesOut, jetAccelerationOut] = fcn(u, jetIntensities, jetDerivatives, Config)
jetDerivativesOut = zeros(4,1);
jetAccelerationOut = zeros(4,1);
for i=1:4
    state = [jetIntensities(i), jetDerivatives(i)];
    x = jetModel.get_xDot(state, Config.jet.coeff(i,:), u(i));
    jetDerivativesOut(i) = x(1);
    jetAccelerationOut(i) = x(2);
end
end

== matlab function FLYING CONTROLLER (CORE) V2.5/Flying State Machine/Compute Gains And References/Trajectory Generator/Compute CoM and Base Rotation References ==
  data: posCoM_init input double; w_R_b_init input double; moveFront input double; pos_vel_acc_jerk_CoM_des output double; moveLateral input double; moveUpDown input double; rotateRoll input double; rotatePitch input double; rotateYaw input double; turbo_mode input double; goLandingPos input double; feetContactIsActive input double; oneFootIsInContact input double; t input double; Config parameter double; rot_vel_acc_jerk_base_des output double
function [pos_vel_acc_jerk_CoM_des, rot_vel_acc_jerk_base_des] = ...
             computeReferencesBaseAndCoMFCN(posCoM_init, w_R_b_init, moveFront, moveLateral, moveUpDown, rotateRoll, rotatePitch, ...
                                            rotateYaw, turbo_mode, goLandingPos, feetContactIsActive, oneFootIsInContact, t, Config)
                                     
    [pos_vel_acc_jerk_CoM_des, rot_vel_acc_jerk_base_des] = ...
        computeReferencesBaseAndCoM(posCoM_init, w_R_b_init, moveFront, moveLateral, moveUpDown, rotateRoll, rotatePitch, ...
                                    rotateYaw, turbo_mode, goLandingPos, feetContactIsActive, oneFootIsInContact, t, Config);
end

== matlab function FLYING CONTROLLER (CORE) V2.5/Flying State Machine/Compute Gains And References/Trajectory Generator/Detect Robot Movement Request From Joystick ==
  data: joyAxes input double; moveFront output double; moveLateral output double; moveUpDown output double; rotateRoll output double; rotatePitch output double; joyButtons input double; rotateYaw output double; turbo_mode output double; goLandingPos output double
function [moveFront, moveLateral, moveUpDown, rotateRoll, rotatePitch, rotateYaw, turbo_mode, goLandingPos] = detectMovementsFromJoystickFCN(joyAxes,joyButtons)

    [moveFront, moveLateral, moveUpDown, rotateRoll, rotatePitch, rotateYaw, turbo_mode, goLandingPos] = detectMovementsFromJoystick(joyAxes,joyButtons);
end

== matlab function iRonCub/Forward Dynamics/old_simulator_subsystem/Dynamics and Kinematics/Kinematic Quantities/Compute Thrusts Axes and Arms/Thrust Axes and Arms ==
  data: w_H_J1 input double; matrixOfJetsAxes output double; w_H_J2 input double; w_H_J3 input double; w_H_J4 input double; posCoM input double; matrixOfJetsArms output double; Config parameter double
function [matrixOfJetsAxes, matrixOfJetsArms] = computeJetsAxesAndArmsFCN(w_H_J1, w_H_J2, w_H_J3, w_H_J4, posCoM, Config)

    [matrixOfJetsAxes, matrixOfJetsArms] = computeJetsAxesAndArms(w_H_J1, w_H_J2, w_H_J3, w_H_J4, posCoM, Config);
end

== matlab function FLYING CONTROLLER (CORE) V2.5/Flying State Machine/Compute Gains And References/Smooth CoM and Base References/Smooth Reference Orientations/Rotational PID Controller/Compute Rotation Matrix Derivative ==
  data: gainSmoothingBaseRot input double; w_R_b_des input double; w_R_b input double; b_omega_b output double; RDot output double
function [b_omega_b, RDot] = rotationDerivativeFromAngVelFCN(gainSmoothingBaseRot, w_R_b_des, w_R_b)
                                                                                                                                                            
    % Rotational PID: 
    %
    % w_R_b_des = reference rotation (may be discontinuous)
    % 
    % b_omega_b = control input for the rotational PID. The angular velocity
    %             is expressed w.r.t. a frame attached to the link, i.e. it 
    %             is expressed in the "body" frame (b).
    % 
    % Kp        = control gain
    %
    % w_R_b     = smooth base rotation
    %
    b_omega_b_des       = zeros(3,1);
    Kp                  = gainSmoothingBaseRot;
    b_omega_b           = rotationalPID_bodyVelocity(w_R_b, w_R_b_des, b_omega_b_des, Kp);
                      
    % compute the rotation matrix derivative given the angular velocity in body frame
    RDot                = rotationDerivativeFromBodyAngVel(b_omega_b, w_R_b); 
end

== matlab function iRonCub/Forward Dynamics/old_simulator_subsystem/Compute generalized external wrench and jet thrust/Compute generalized jet wrench/compute_jet_wrenches  ==
  data: matrix_of_jet_axis input double; wrenches_vector output double; jet_intensities input double
function wrenches_vector = compute_jet_wrenches(matrix_of_jet_axis, jet_intensities)
dim_wrench = 6;
num_jets = 4;

% the jets produce pure force (no momentum)
% the wrench is a 6dim vector [Fx, Fy, Fz, 0, 0, 0].transpose

wrenches_vector = zeros(dim_wrench*num_jets, 1);
for i=0:(num_jets-1)
    wrenches_vector(dim_wrench*i + 1: dim_wrench*i + dim_wrench/2) = matrix_of_jet_axis(:,i+1)*jet_intensities(i+1);
end
